simulink model "S1"  (R2023b)
settings: Solver=FixedStepAuto  StartTime=0.0  StopTime=Time_data-Step_T  FixedStep=Step_T  RelTol=1e-3
InitFcn:
  | run("P_sim.m")
values from neighbouring files (symbols this model uses):
  T = 1    [P_sim.m]
  x_1_0 = 0.5    [P_sim.m]
  x_2_0 = -0.5    [P_sim.m]
settings Model: Creator=admin  LastModifiedBy=admin

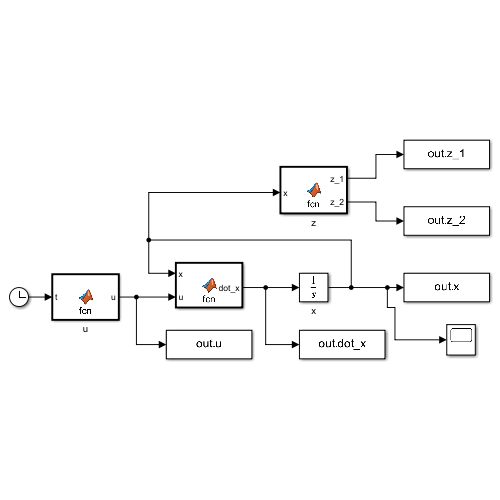
[thumbnail: Simulink's stored preview of the top-level diagram]
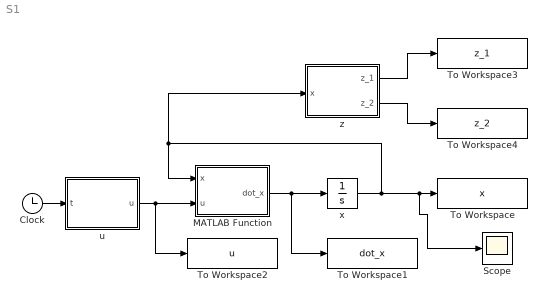
== system S1 ==
  Clock : Clock
  MATLAB Function : MATLAB Function  TreatAsAtomicUnit=on
  Scope : Scope
  To Workspace : ToWorkspace  VariableName=x  SaveFormat=Timeseries  SampleTime=T
  To Workspace1 : ToWorkspace  VariableName=dot_x  SaveFormat=Timeseries  SampleTime=T
  To Workspace2 : ToWorkspace  VariableName=u  SaveFormat=Timeseries  SampleTime=T
  To Workspace3 : ToWorkspace  VariableName=z_1  SaveFormat=Timeseries  SampleTime=T
  To Workspace4 : ToWorkspace  VariableName=z_2  SaveFormat=Timeseries  SampleTime=T
  u : MATLAB Function  TreatAsAtomicUnit=on
  x : Integrator  InitialCondition=[x_1_0;x_2_0]
  z : MATLAB Function  TreatAsAtomicUnit=on
  wires:
  MATLAB Function/1(dot_x) -> To Workspace1/1, x/1
  x/1 -> Scope/1, To Workspace/1, MATLAB Function/1(x), z/1(x)
  u/1(u) -> To Workspace2/1, MATLAB Function/2(u)
  Clock/1 -> u/1(t)
  z/1(z_1) -> To Workspace3/1
  z/2(z_2) -> To Workspace4/1

== matlab function S1/MATLAB Function ==
  data: x input; dot_x output; u input
function dot_x  = fcn(x,u)

x_1 = x(1);
x_2 = x(2);

dot_x_1 = x_2-2*x_1;
dot_x_2 = u+3*x_1-x_1*x_2+x_2^2;

dot_x = [dot_x_1;dot_x_2];

== matlab function S1/z ==
  data: x input; z_1 output; z_2 output
function [z_1,z_2]  = fcn(x)

x_1 = x(1);
x_2 = x(2);

z_1 = [x_1;x_1^2];
z_2 = [x_1;x_2;x_1*x_2;x_1^2;x_2^2];

== matlab function S1/u ==
  data: t input; u output
function u  = fcn(t)

u = -0.5+0.1*t;
